simulink model "formation_planner_exp_cs"  (R2022b)
settings: Solver=ode5  StartTime=0.0  StopTime=80  FixedStep=1/1000  RelTol=1e-3
PreLoadFcn:
  | mbxruntime.callbacks.PreLoadFcn(bdroot);
PostLoadFcn:
  | mbxruntime.callbacks.PostLoadFcn(bdroot);
InitFcn:
  | mbxruntime.callbacks.InitFcn(bdroot);
StartFcn:
  | mbxruntime.callbacks.StartFcn(bdroot);
StopFcn:
  | mbxruntime.callbacks.StopFcn(bdroot);
model workspace (MAT data in the model file):
  mbox_table : object (value not decoded)
  model_closed = 0
  sim_status = 0
values from neighbouring files (symbols this model uses):
  c_factor = 43.75    [emplanner_init.m]
  car1_s = -10    [emplanner_init.m]
  car2_s = -20    [emplanner_init.m]
  cf = -175016    [emplanner_init.m]
  cr = -130634    [emplanner_init.m]
  KD_PID_distance = 0.0    (= 0)    [emplanner_init.m]
  KD_PID_speed = 0    [emplanner_init.m]
  KI_PID_distance = 0.0    (= 0)    [emplanner_init.m]
  KI_PID_speed = 0    [emplanner_init.m]
  KP_PID_distance = 0.5    [emplanner_init.m]
  KP_PID_speed = 1.8    [emplanner_init.m]
  la = 1.265    [emplanner_init.m]
  lb = 2.947-1.265    (= 1.682)    [emplanner_init.m]
  leader_global_kappa = global_kappa    [kappa.m]    (also in leader_global_path.mat = [0 0 0 0 0 0 0 0 0 0 0 0 ... (801 elements, 801x1)])
  leader_global_path_x = x_orgin.Data    [kappa.m]    (also in leader_global_path.mat = [2.22044604925e-16 0.999382255067 1.99750536558 2.9943522493)
  leader_global_path_y = y.Data    [kappa.m]    (also in leader_global_path.mat = [2 2 2 2 2 2 2 2 2 2 2 2 ... (801 elements, 801x1)])
  leader_global_yaw = yaw.Data    [kappa.m]    (also in leader_global_path.mat = [0 0 0 0 0 0 0 0 0 0 0 0 ... (801 elements, 801x1)])
  LQR_K1 = k(:,1)'    [emplanner_init.m]
  LQR_K2 = k(:,2)'    [emplanner_init.m]
  LQR_K3 = k(:,3)'    [emplanner_init.m]
  LQR_K4 = k(:,4)'    [emplanner_init.m]
  m = 2020    [emplanner_init.m]
  rack_displacement = [-39.14 , -37.2 , -35.29 , -33.43 , -31.6 , -29.81 , -28.06 , -26.34 , -24.66 ,      -23.01 , -21.38 , -19.79 , -18.23 , -16.69 , -15.18 , -13.7 , -12.23 , -10.8 , -9.38 , -7.98 ,     -6.61 , -5.25 , -3.91 , -2.59 , -1.29 , 0 , 1.27 , 2.54 , 3.78 , 5.02 , 6.24 , 7.46 , 8.66 ,      9.86 , 11.05 , 12.24 , 13.41 , 14.59 , 15.76 , 16.92 , 18.09 , 19.25 , 20.42 , 21.59 , 22.76 ,      23.93 , 25.11 , 26 ...(+26 chars)    [emplanner_init.m]
  right_wheel_ground = [-70 ,-67.2 , -64.4 , -61.6 , -58.8 , -56 , -53.2 , -50.4 , -47.6 , -44.8 , -42 ,      -39.2 , -36.4 , -33.6 , -30.8 , -28 , -25.2 , -22.4 , -19.6 , -16.8 , -14 , -11.2 , -8.4 , -5.6 ,      -2.8 , 0 , 2.8 , 5.6 , 8.4 , 11.2 , 14 , 16.8 , 19.6 , 22.4 , 25.2 , 28 , 30.8 , 33.6 , 36.4 ,      39.2 , 42 , 44.8 , 47.6 , 50.4 , 53.2 , 56 , 58.8 , 61.6 , 64.4 , 67.2 , 70 ]    [emplanner_init.m]
  vx_break_point = zeros(1,5000)    [emplanner_init.m]
undefined symbols (not defined in the file or in its folder): aubr, car1_global_kappa, car1_global_path_x, car1_global_path_y, car1_global_yaw, car2_global_kappa, car2_global_path_x, car2_global_path_y, car2_global_yaw, DiscIntNeverNeededParam, tablebr, vubr, warningInitialVelocity, x0
libraries: PreScanSimulinkLibrary x65, simulink x19, simulink_extras x14, Solver_SF x2
(part 15 of 31)

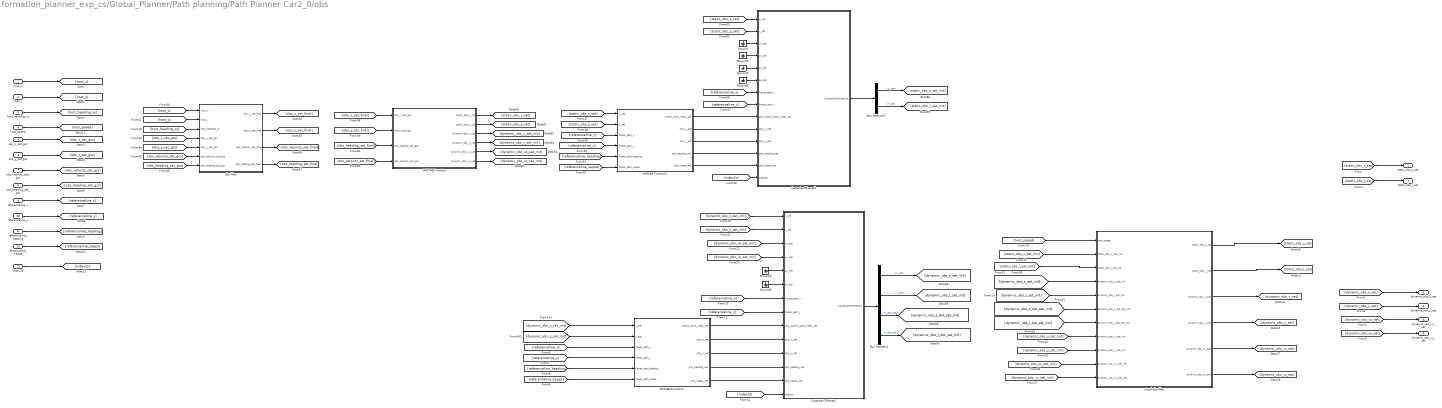
== system formation_planner_exp_cs/Global_Planner/Path planning/Path Planner Car2_0/obs ==
  host_x : Inport
  host_y : Inport  Port=2
  host_heading_xy : Inport  Port=3
  host_speed : Inport  Port=4
  obs_x_set_gcs : Inport  Port=5
  obs_y_set_gcs : Inport  Port=6
  obs_velocity_set_gcs : Inport  Port=7
  obs_heading_set_gcs : Inport  Port=8
  referenceline_x : Inport  Port=9
  referenceline_y : Inport  Port=10
  referenceline_heading : Inport  Port=11
  referenceline_kappa : Inport  Port=12
  index2s : Inport  Port=13
  Bus Selector1 : BusSelector  OutputSignals=s_set,l_set,s_dot_set,l_dot_set
  Bus Selector5 : BusSelector  OutputSignals=s_set,l_set
  Cartesian2Frenet1 : Subsystem
  Cartesian2Frenet2 : Subsystem
  Ground{,1..5} (6 alike) : Ground
  MATLAB Function : MATLAB Function  TreatAsAtomicUnit=on
  MATLAB Function1 : MATLAB Function  TreatAsAtomicUnit=on
  MATLAB Function2 : MATLAB Function  TreatAsAtomicUnit=on
  obs filter : MATLAB Function  TreatAsAtomicUnit=on
  visual obs filter : MATLAB Function  TreatAsAtomicUnit=on
  static_obs_s_set : Outport
  static_obs_l_set : Outport  Port=2
  dynamic_obs_x_set : Outport  Port=3
  dynamic_obs_y_set : Outport  Port=4
  dynamic_obs_vx_set : Outport  Port=5
  dynamic_obs_vy_set : Outport  Port=6
  wires:
  Ground3/1 -> Cartesian2Frenet1/6(ay_set)
  [obs_x_set_gcs] -> obs filter/4(obs_x_set_gcs)
  [index2s] -> Cartesian2Frenet1/14(index2s)
  [referenceline_y] -> Cartesian2Frenet1/8(frenet_path_y)
  MATLAB Function2/5(proj_kappa_set) -> Cartesian2Frenet1/13(proj_kappa_set)
  MATLAB Function2/4(proj_heading_set) -> Cartesian2Frenet1/12(proj_heading_set)
  [referenceline_x] -> MATLAB Function2/3(frenet_path_x)
  Ground2/1 -> Cartesian2Frenet1/5(ax_set)
  obs filter/1(obs_x_set_final) -> [obs_x_set_final]
  obs filter/4(obs_heading_set_final) -> [obs_heading_set_final]
  [host_heading_xy] -> obs filter/3(host_heading_xy)
  MATLAB Function/5(dynamic_obs_vx_set) -> [dynamic_obs_vx_set_init]
  [obs_y_set_final] -> MATLAB Function/2(obs_y_set_gcs)
  MATLAB Function/6(dynamic_obs_vy_set) -> [dynamic_obs_vy_set_init]
  [referenceline_y] -> MATLAB Function2/4(frenet_path_y)
  obs filter/3(obs_velocity_set_final) -> [obs_velocity_set_final]
  MATLAB Function/1(static_obs_x_set) -> [static_obs_x_set]
  [obs_heading_set_gcs] -> obs filter/7(obs_heading_set_gcs)
  [referenceline_kappa] -> MATLAB Function2/6(frenet_path_kappa)
  [static_obs_x_set] -> Cartesian2Frenet1/1(x_set)
  [static_obs_y_set] -> MATLAB Function2/2(y_set)
  [referenceline_x] -> Cartesian2Frenet1/7(frenet_path_x)
  Ground1/1 -> Cartesian2Frenet1/4(vy_set)
  [obs_x_set_final] -> MATLAB Function/1(obs_x_set_gcs)
  [obs_velocity_set_gcs] -> obs filter/6(obs_velocity_set_gcs)
  [host_y] -> obs filter/2(host_y)
  Bus Selector5/2 -> [static_obs_l_set_init]  "<l_set>"
  [referenceline_heading] -> MATLAB Function2/5(frenet_path_heading)
  obs filter/2(obs_y_set_final) -> [obs_y_set_final]
  Bus Selector5/1 -> [static_obs_s_set_init]  "<s_set>"
  MATLAB Function/3(dynamic_obs_x_set) -> [dynamic_obs_x_set_init]
  MATLAB Function2/2(proj_x_set) -> Cartesian2Frenet1/10(proj_x_set)
  Ground/1 -> Cartesian2Frenet1/3(vx_set)
  MATLAB Function2/3(proj_y_set) -> Cartesian2Frenet1/11(proj_y_set)
  MATLAB Function/4(dynamic_obs_y_set) -> [dynamic_obs_y_set_init]
  MATLAB Function2/1(match_point_index_set) -> Cartesian2Frenet1/9(proj_match_point_index_set)
  [host_x] -> obs filter/1(host_x)
  [obs_y_set_gcs] -> obs filter/5(obs_y_set_gcs)
  Cartesian2Frenet1/1(Cartesian2FrenetOut) -> Bus Selector5/1
  [static_obs_x_set] -> MATLAB Function2/1(x_set)
  MATLAB Function/2(static_obs_y_set) -> [static_obs_y_set]
  [static_obs_y_set] -> Cartesian2Frenet1/2(y_set)
  host_x/1 -> [host_x]
  host_y/1 -> [host_y]
  host_heading_xy/1 -> [host_heading_xy]
  obs_x_set_gcs/1 -> [obs_x_set_gcs]
  obs_y_set_gcs/1 -> [obs_y_set_gcs]
  obs_velocity_set_gcs/1 -> [obs_velocity_set_gcs]
  obs_heading_set_gcs/1 -> [obs_heading_set_gcs]
  referenceline_x/1 -> [referenceline_x]
  referenceline_y/1 -> [referenceline_y]
  referenceline_heading/1 -> [referenceline_heading]
  referenceline_kappa/1 -> [referenceline_kappa]
  index2s/1 -> [index2s]
  [static_obs_s_set] -> static_obs_s_set/1
  [static_obs_l_set] -> static_obs_l_set/1
  [dynamic_obs_vy_set] -> dynamic_obs_vy_set/1
  [dynamic_obs_vx_set] -> dynamic_obs_vx_set/1
  [dynamic_obs_y_set] -> dynamic_obs_y_set/1
  [dynamic_obs_x_set] -> dynamic_obs_x_set/1
  [obs_velocity_set_final] -> MATLAB Function/4(obs_velocity_set_gcs)
  [obs_heading_set_final] -> MATLAB Function/3(obs_heading_set_gcs)
  [referenceline_x] -> Cartesian2Frenet2/7(frenet_path_x)
  Bus Selector1/1 -> [dynamic_obs_s_set_init]  "<s_set>"
  Ground4/1 -> Cartesian2Frenet2/5(ax_set)
  MATLAB Function1/2(proj_x_set) -> Cartesian2Frenet2/10(proj_x_set)
  Bus Selector1/2 -> [dynamic_obs_l_set_init]  "<l_set>"
  [dynamic_obs_vx_set_init] -> Cartesian2Frenet2/3(vx_set)
  [dynamic_obs_y_set_init] -> MATLAB Function1/2(y_set)
  Bus Selector1/4 -> [dynamic_obs_l_dot_set_init]  "<l_dot_set>"
  [referenceline_kappa] -> MATLAB Function1/6(frenet_path_kappa)
  Cartesian2Frenet2/1(Cartesian2FrenetOut) -> Bus Selector1/1
  MATLAB Function1/3(proj_y_set) -> Cartesian2Frenet2/11(proj_y_set)
  [index2s] -> Cartesian2Frenet2/14(index2s)
  MATLAB Function1/1(match_point_index_set) -> Cartesian2Frenet2/9(proj_match_point_index_set)
  [referenceline_heading] -> MATLAB Function1/5(frenet_path_heading)
  [dynamic_obs_y_set_init] -> Cartesian2Frenet2/2(y_set)
  [dynamic_obs_vy_set_init] -> Cartesian2Frenet2/4(vy_set)
  [referenceline_y] -> Cartesian2Frenet2/8(frenet_path_y)
  [referenceline_y] -> MATLAB Function1/4(frenet_path_y)
  [dynamic_obs_x_set_init] -> MATLAB Function1/1(x_set)
  Bus Selector1/3 -> [dynamic_obs_s_dot_set_init]  "<s_dot_set>"
  MATLAB Function1/4(proj_heading_set) -> Cartesian2Frenet2/12(proj_heading_set)
  Ground5/1 -> Cartesian2Frenet2/6(ay_set)
  [dynamic_obs_x_set_init] -> Cartesian2Frenet2/1(x_set)
  MATLAB Function1/5(proj_kappa_set) -> Cartesian2Frenet2/13(proj_kappa_set)
  [referenceline_x] -> MATLAB Function1/3(frenet_path_x)
  [dynamic_obs_s_dot_set_init] -> visual obs filter/6(dynamic_obs_s_dot_set_init)
  [dynamic_obs_l_dot_set_init] -> visual obs filter/7(dynamic_obs_l_dot_set_init)
  [dynamic_obs_s_set_init] -> visual obs filter/4(dynamic_obs_s_set_init)
  [dynamic_obs_l_set_init] -> visual obs filter/5(dynamic_obs_l_set_init)
  [static_obs_s_set_init] -> visual obs filter/2(static_obs_s_set_init)
  [static_obs_l_set_init] -> visual obs filter/3(static_obs_l_set_init)
  host_speed/1 -> [host_speed]
  [host_speed] -> visual obs filter/1(host_speed)
  visual obs filter/6(dynamic_obs_vy_set) -> [dynamic_obs_vy_set]
  visual obs filter/5(dynamic_obs_vx_set) -> [dynamic_obs_vx_set]
  visual obs filter/4(dynamic_obs_y_set) -> [dynamic_obs_y_set]
  visual obs filter/1(static_obs_s_set) -> [static_obs_s_set]
  visual obs filter/2(static_obs_l_set) -> [static_obs_l_set]
  visual obs filter/3(dynamic_obs_x_set) -> [dynamic_obs_x_set]
  [dynamic_obs_x_set_init] -> visual obs filter/8(dynamic_obs_x_set_init)
  [dynamic_obs_y_set_init] -> visual obs filter/9(dynamic_obs_y_set_init)
  [dynamic_obs_vx_set_init] -> visual obs filter/10(dynamic_obs_vx_set_init)
  [dynamic_obs_vy_set_init] -> visual obs filter/11(dynamic_obs_vy_set_init)

== system formation_planner_exp_cs/Global_Planner/Path planning/Path Planner Car2_0/path decision task ==
  static_obs_s_set : Inport
  static_obs_l_set : Inport  Port=2
  plan_start_s : Inport  Port=3
  plan_start_l : Inport  Port=4
  plan_start_dl : Inport  Port=5
  plan_start_ddl : Inport  Port=6
  dp_cost_collision : Inport  Port=7
  dp_cost_dl : Inport  Port=8
  dp_cost_ddl : Inport  Port=9
  dp_cost_dddl : Inport  Port=10
  dp_cost_ref : Inport  Port=11
  dp_row : Inport  Port=12
  dp_col : Inport  Port=13
  dp_sample_s : Inport  Port=14
  dp_sample_l : Inport  Port=15
  increase DP path nodes : MATLAB Function  TreatAsAtomicUnit=on
  path decision with dynamic planning(dp) : MATLAB Function  TreatAsAtomicUnit=on
  dp_path_s_final : Outport
  dp_path_l_final : Outport  Port=2
  dp_path_dl_final : Outport  Port=3
  dp_path_ddl_final : Outport  Port=4
  wires:
  [plan_start_s] -> path decision with dynamic planning(dp)/3(plan_start_s)
  path decision with dynamic planning(dp)/1(dp_path_s) -> [dp_path_s_init]
  increase DP path nodes/2(dp_path_l_final) -> [dp_path_l_final]
  [static_obs_l_set] -> path decision with dynamic planning(dp)/2(obs_l_set)
  [plan_start_ddl] -> path decision with dynamic planning(dp)/6(plan_start_dll)
  [plan_start_l] -> path decision with dynamic planning(dp)/4(plan_start_l)
  [static_obs_s_set] -> path decision with dynamic planning(dp)/1(obs_s_set)
  [plan_start_dl] -> increase DP path nodes/5(plan_start_dl)
  increase DP path nodes/4(dp_path_ddl_final) -> [dp_path_ddl_final]
  increase DP path nodes/1(dp_path_s_final) -> [dp_path_s_final]
  increase DP path nodes/3(dp_path_dl_final) -> [dp_path_dl_final]
  path decision with dynamic planning(dp)/2(dp_path_l) -> [dp_path_l_init]
  [plan_start_l] -> increase DP path nodes/4(plan_start_l)
  [plan_start_ddl] -> increase DP path nodes/6(plan_start_ddl)
  [plan_start_dl] -> path decision with dynamic planning(dp)/5(plan_start_dl)
  [plan_start_s] -> increase DP path nodes/3(plan_start_s)
  [dp_path_l_init] -> increase DP path nodes/2(dp_path_l_init)
  [dp_path_s_init] -> increase DP path nodes/1(dp_path_s_init)
  static_obs_s_set/1 -> [static_obs_s_set]
  static_obs_l_set/1 -> [static_obs_l_set]
  plan_start_s/1 -> [plan_start_s]
  plan_start_l/1 -> [plan_start_l]
  plan_start_dl/1 -> [plan_start_dl]
  plan_start_ddl/1 -> [plan_start_ddl]
  [dp_path_s_final] -> dp_path_s_final/1
  [dp_path_l_final] -> dp_path_l_final/1
  [dp_path_dl_final] -> dp_path_dl_final/1
  [dp_path_ddl_final] -> dp_path_ddl_final/1
  [dp_cost_collision] -> path decision with dynamic planning(dp)/7(w_cost_collision)
  [dp_cost_dl] -> path decision with dynamic planning(dp)/8(w_cost_smooth_dl)
  [dp_cost_ddl] -> path decision with dynamic planning(dp)/9(w_cost_smooth_ddl)
  [dp_cost_dddl] -> path decision with dynamic planning(dp)/10(w_cost_smooth_dddl)
  [dp_cost_ref] -> path decision with dynamic planning(dp)/11(w_cost_ref)
  [dp_row] -> path decision with dynamic planning(dp)/12(row)
  [dp_col] -> path decision with dynamic planning(dp)/13(col)
  [dp_sample_s] -> path decision with dynamic planning(dp)/14(sample_s)
  [dp_sample_l] -> path decision with dynamic planning(dp)/15(sample_l)
  dp_cost_dl/1 -> [dp_cost_dl]
  dp_cost_ddl/1 -> [dp_cost_ddl]
  dp_cost_dddl/1 -> [dp_cost_dddl]
  dp_cost_ref/1 -> [dp_cost_ref]
  dp_row/1 -> [dp_row]
  dp_col/1 -> [dp_col]
  dp_sample_l/1 -> [dp_sample_l]
  dp_sample_s/1 -> [dp_sample_s]
  dp_cost_collision/1 -> [dp_cost_collision]

== system formation_planner_exp_cs/Global_Planner/Path planning/Path Planner Car2_0/path planning task ==
  dp_path_s_final : Inport
  dp_path_l_final : Inport  Port=2
  static_obs_s_set : Inport  Port=3
  static_obs_l_set : Inport  Port=4
  plan_start_s : Inport  Port=5
  plan_start_l : Inport  Port=6
  plan_start_dl : Inport  Port=7
  plan_start_ddl : Inport  Port=8
  qp_cost_l : Inport  Port=9
  qp_cost_dl : Inport  Port=10
  qp_cost_ddl : Inport  Port=11
  qp_cost_dddl : Inport  Port=12
  qp_cost_centre : Inport  Port=13
  qp_cost_endl : Inport  Port=14
  qp_cost_end_dl : Inport  Port=15
  qp_cost_end_ddl : Inport  Port=16
  host_d1 : Inport  Port=17
  host_d2 : Inport  Port=18
  host_w : Inport  Port=19
  delta_dl_max : Inport  Port=20
  delta_ddl_max : Inport  Port=21
  Constant10 : Constant  Value=5
  Constant11 : Constant  Value=3
  MATLAB Function : MATLAB Function  TreatAsAtomicUnit=on
  generate convex space : MATLAB Function  TreatAsAtomicUnit=on
  path planning with quadratic programming (qp) : MATLAB Function  TreatAsAtomicUnit=on
  qp_path_s_final : Outport
  qp_path_l_final : Outport  Port=2
  qp_path_dl_final : Outport  Port=3
  qp_path_ddl_final : Outport  Port=4
  wires:
  generate convex space/2(l_max) -> [l_max]
  Constant11/1 -> generate convex space/6(static_obs_width)
  Constant10/1 -> generate convex space/5(static_obs_length)
  [static_obs_l_set] -> generate convex space/4(static_obs_l_set)
  [dp_path_s_final] -> generate convex space/1(dp_path_s)
  [plan_start_l] -> path planning with quadratic programming (qp)/15(plan_start_l)
  generate convex space/1(l_min) -> [l_min]
  [static_obs_s_set] -> generate convex space/3(static_obs_s_set)
  [dp_path_l_final] -> generate convex space/2(dp_path_l)
  [plan_start_dl] -> path planning with quadratic programming (qp)/16(plan_start_dl)
  [l_max] -> path planning with quadratic programming (qp)/2(l_max)
  [l_min] -> path planning with quadratic programming (qp)/1(l_min)
  [plan_start_ddl] -> path planning with quadratic programming (qp)/17(plan_start_ddl)
  dp_path_s_final/1 -> [dp_path_s_final]
  dp_path_l_final/1 -> [dp_path_l_final]
  static_obs_s_set/1 -> [static_obs_s_set]
  static_obs_l_set/1 -> [static_obs_l_set]
  plan_start_l/1 -> [plan_start_l]
  plan_start_dl/1 -> [plan_start_dl]
  plan_start_ddl/1 -> [plan_start_ddl]
  [qp_cost_l] -> path planning with quadratic programming (qp)/3(w_cost_l)
  [qp_cost_dl] -> path planning with quadratic programming (qp)/4(w_cost_dl)
  [qp_cost_ddl] -> path planning with quadratic programming (qp)/5(w_cost_ddl)
  [qp_cost_dddl] -> path planning with quadratic programming (qp)/6(w_cost_dddl)
  [qp_cost_centre] -> path planning with quadratic programming (qp)/7(w_cost_centre)
  [qp_cost_endl] -> path planning with quadratic programming (qp)/8(w_cost_end_l)
  [qp_cost_end_dl] -> path planning with quadratic programming (qp)/9(w_cost_end_dl)
  [qp_cost_end_ddl] -> path planning with quadratic programming (qp)/10(w_cost_end_ddl)
  [host_d1] -> path planning with quadratic programming (qp)/11(host_d1)
  [host_d2] -> path planning with quadratic programming (qp)/12(host_d2)
  [host_w] -> path planning with quadratic programming (qp)/13(host_w)
  qp_cost_l/1 -> [qp_cost_l]
  qp_cost_dl/1 -> [qp_cost_dl]
  qp_cost_ddl/1 -> [qp_cost_ddl]
  qp_cost_dddl/1 -> [qp_cost_dddl]
  qp_cost_centre/1 -> [qp_cost_centre]
  qp_cost_endl/1 -> [qp_cost_endl]
  qp_cost_end_dl/1 -> [qp_cost_end_dl]
  qp_cost_end_ddl/1 -> [qp_cost_end_ddl]
  host_d1/1 -> [host_d1]
  host_d2/1 -> [host_d2]
  host_w/1 -> [host_w]
  [delta_dl_max] -> path planning with quadratic programming (qp)/18(delta_dl_max)
  [delta_ddl_max] -> path planning with quadratic programming (qp)/19(delta_ddl_max)
  delta_dl_max/1 -> [delta_dl_max]
  delta_ddl_max/1 -> [delta_ddl_max]
  plan_start_s/1 -> [plan_start_s]
  [plan_start_s] -> path planning with quadratic programming (qp)/14(plan_start_s)
  MATLAB Function/1(qp_path_s_final) -> [qp_path_s_final]
  MATLAB Function/3(qp_path_dl_final) -> [qp_path_dl_final]
  [qp_path_s] -> MATLAB Function/1(qp_path_s)
  [qp_path_ddl] -> MATLAB Function/4(qp_path_ddl)
  MATLAB Function/2(qp_path_l_final) -> [qp_path_l_final]
  [qp_path_dl] -> MATLAB Function/3(qp_path_dl)
  MATLAB Function/4(qp_path_ddl_final) -> [qp_path_ddl_final]
  [qp_path_l] -> MATLAB Function/2(qp_path_l)
  [qp_path_s_final] -> qp_path_s_final/1
  [qp_path_l_final] -> qp_path_l_final/1
  [qp_path_dl_final] -> qp_path_dl_final/1
  [qp_path_ddl_final] -> qp_path_ddl_final/1
  path planning with quadratic programming (qp)/1(qp_path_s) -> [qp_path_s]
  path planning with quadratic programming (qp)/2(qp_path_l) -> [qp_path_l]
  path planning with quadratic programming (qp)/3(qp_path_dl) -> [qp_path_dl]
  path planning with quadratic programming (qp)/4(qp_path_ddl) -> [qp_path_ddl]

== system formation_planner_exp_cs/Global_Planner/Path planning/Planner Car1/Cartesian2Frenet ==
  x_set : Inport
  y_set : Inport  Port=2
  vx_set : Inport  Port=3
  vy_set : Inport  Port=4
  ax_set : Inport  Port=5
  ay_set : Inport  Port=6
  frenet_path_x : Inport  Port=7
  frenet_path_y : Inport  Port=8
  proj_match_point_index_set : Inport  Port=9
  proj_x_set : Inport  Port=10
  proj_y_set : Inport  Port=11
  proj_heading_set : Inport  Port=12
  proj_kappa_set : Inport  Port=13
  index2s : Inport  Port=14
  Bus Creator : BusCreator  Inputs=8
  MATLAB Function : MATLAB Function  TreatAsAtomicUnit=on
  MATLAB Function1 : MATLAB Function  TreatAsAtomicUnit=on
  MATLAB Function2 : MATLAB Function  TreatAsAtomicUnit=on
  Cartesian2FrenetOut : Outport
  wires:
  Bus Creator/1 -> Cartesian2FrenetOut/1
  [ddl_set] -> Bus Creator/8  "ddl_set"
  [l_dot2_set] -> Bus Creator/7  "l_dot2_set"
  [s_dot2_set] -> Bus Creator/6  "s_dot2_set"
  [dl_set] -> Bus Creator/5  "dl_set"
  [l_dot_set] -> Bus Creator/4  "l_dot_set"
  [s_dot_set] -> Bus Creator/3  "s_dot_set"
  [l_set] -> Bus Creator/2  "l_set"
  [s_set] -> Bus Creator/1  "s_set"
  MATLAB Function2/3(ddl_set) -> [ddl_set]
  MATLAB Function2/2(l_dot2_set) -> [l_dot2_set]
  MATLAB Function2/1(s_dot2_set) -> [s_dot2_set]
  [dl_set] -> MATLAB Function2/7(dl_set)
  [s_dot_set] -> MATLAB Function2/6(s_dot_set)
  MATLAB Function1/3(dl_set) -> [dl_set]
  MATLAB Function1/2(l_dot_set) -> [l_dot_set]
  MATLAB Function1/1(s_dot_set) -> [s_dot_set]
  [l_set] -> MATLAB Function2/5(l_set)
  [proj_kappa_set] -> MATLAB Function2/4(proj_kappa_set)
  [proj_heading_set] -> MATLAB Function2/3(proj_heading_set)
  [ay_set] -> MATLAB Function2/2(ay_set)
  [ax_set] -> MATLAB Function2/1(ax_set)
  [proj_kappa_set] -> MATLAB Function1/5(proj_kappa_set)
  [proj_heading_set] -> MATLAB Function1/4(proj_heading_set)
  [vy_set] -> MATLAB Function1/3(vy_set)
  [vx_set] -> MATLAB Function1/2(vx_set)
  [l_set] -> MATLAB Function1/1(l_set)
  MATLAB Function/2(l_set) -> [l_set]
  MATLAB Function/1(s_set) -> [s_set]
  [index2s] -> MATLAB Function/9(index2s)
  [proj_heading_set] -> MATLAB Function/7(proj_heading_set)
  [proj_y_set] -> MATLAB Function/6(proj_y_set)
  [proj_match_point_index_set] -> MATLAB Function/8(proj_match_point_index_set)
  [proj_x_set] -> MATLAB Function/5(proj_x_set)
  [frenet_path_y] -> MATLAB Function/4(frenet_path_y)
  [frenet_path_x] -> MATLAB Function/3(frenet_path_x)
  [y_set] -> MATLAB Function/2(y_set)
  [x_set] -> MATLAB Function/1(x_set)
  index2s/1 -> [index2s]
  proj_kappa_set/1 -> [proj_kappa_set]
  proj_heading_set/1 -> [proj_heading_set]
  proj_y_set/1 -> [proj_y_set]
  proj_x_set/1 -> [proj_x_set]
  proj_match_point_index_set/1 -> [proj_match_point_index_set]
  frenet_path_y/1 -> [frenet_path_y]
  frenet_path_x/1 -> [frenet_path_x]
  ay_set/1 -> [ay_set]
  ax_set/1 -> [ax_set]
  vy_set/1 -> [vy_set]
  vx_set/1 -> [vx_set]
  y_set/1 -> [y_set]
  x_set/1 -> [x_set]

== system formation_planner_exp_cs/Global_Planner/Path planning/Planner Car1/Cartesian2Frenet1 ==
  x_set : Inport
  y_set : Inport  Port=2
  vx_set : Inport  Port=3
  vy_set : Inport  Port=4
  ax_set : Inport  Port=5
  ay_set : Inport  Port=6
  frenet_path_x : Inport  Port=7
  frenet_path_y : Inport  Port=8
  proj_match_point_index_set : Inport  Port=9
  proj_x_set : Inport  Port=10
  proj_y_set : Inport  Port=11
  proj_heading_set : Inport  Port=12
  proj_kappa_set : Inport  Port=13
  index2s : Inport  Port=14
  Bus Creator : BusCreator  Inputs=8
  From14 : From  Commented=on  GotoTag=ax_set
  From15 : From  Commented=on  GotoTag=ay_set
  From16 : From  Commented=on  GotoTag=proj_heading_set
  From17 : From  Commented=on  GotoTag=proj_kappa_set
  From18 : From  Commented=on  GotoTag=l_set
  From19 : From  Commented=on  GotoTag=s_dot_set
  From20 : From  Commented=on  GotoTag=dl_set
  Goto19 : Goto  Commented=on  GotoTag=s_dot2_set
  Goto20 : Goto  Commented=on  GotoTag=l_dot2_set
  Goto21 : Goto  Commented=on  GotoTag=ddl_set
  MATLAB Function : MATLAB Function  TreatAsAtomicUnit=on
  MATLAB Function1 : MATLAB Function  TreatAsAtomicUnit=on
  MATLAB Function2 : MATLAB Function  Commented=on  TreatAsAtomicUnit=on
  Cartesian2FrenetOut : Outport
  wires:
  x_set/1 -> [x_set]
  y_set/1 -> [y_set]
  vx_set/1 -> [vx_set]
  vy_set/1 -> [vy_set]
  ax_set/1 -> [ax_set]
  ay_set/1 -> [ay_set]
  frenet_path_x/1 -> [frenet_path_x]
  frenet_path_y/1 -> [frenet_path_y]
  proj_match_point_index_set/1 -> [proj_match_point_index_set]
  proj_x_set/1 -> [proj_x_set]
  proj_y_set/1 -> [proj_y_set]
  proj_heading_set/1 -> [proj_heading_set]
  proj_kappa_set/1 -> [proj_kappa_set]
  index2s/1 -> [index2s]
  [x_set] -> MATLAB Function/1(x_set)
  [y_set] -> MATLAB Function/2(y_set)
  [frenet_path_x] -> MATLAB Function/3(frenet_path_x)
  [frenet_path_y] -> MATLAB Function/4(frenet_path_y)
  [proj_x_set] -> MATLAB Function/5(proj_x_set)
  [proj_match_point_index_set] -> MATLAB Function/8(proj_match_point_index_set)
  [proj_y_set] -> MATLAB Function/6(proj_y_set)
  [proj_heading_set] -> MATLAB Function/7(proj_heading_set)
  [index2s] -> MATLAB Function/9(index2s)
  MATLAB Function/1(s_set) -> [s_set]
  MATLAB Function/2(l_set) -> [l_set]
  [l_set] -> MATLAB Function1/1(l_set)
  [vx_set] -> MATLAB Function1/2(vx_set)
  [vy_set] -> MATLAB Function1/3(vy_set)
  [proj_heading_set] -> MATLAB Function1/4(proj_heading_set)
  [proj_kappa_set] -> MATLAB Function1/5(proj_kappa_set)
  From14/1 -> MATLAB Function2/1(ax_set)
  From15/1 -> MATLAB Function2/2(ay_set)
  From16/1 -> MATLAB Function2/3(proj_heading_set)
  From17/1 -> MATLAB Function2/4(proj_kappa_set)
  From18/1 -> MATLAB Function2/5(l_set)
  MATLAB Function1/1(s_dot_set) -> [s_dot_set]
  MATLAB Function1/2(l_dot_set) -> [l_dot_set]
  MATLAB Function1/3(dl_set) -> [dl_set]
  From19/1 -> MATLAB Function2/6(s_dot_set)
  From20/1 -> MATLAB Function2/7(dl_set)
  MATLAB Function2/1(s_dot2_set) -> Goto19/1
  MATLAB Function2/2(l_dot2_set) -> Goto20/1
  MATLAB Function2/3(ddl_set) -> Goto21/1
  [s_set] -> Bus Creator/1  "s_set"
  [l_set] -> Bus Creator/2  "l_set"
  [s_dot_set] -> Bus Creator/3  "s_dot_set"
  [l_dot_set] -> Bus Creator/4  "l_dot_set"
  [dl_set] -> Bus Creator/5  "dl_set"
  [s_dot2_set] -> Bus Creator/6  "s_dot2_set"
  [l_dot2_set] -> Bus Creator/7  "l_dot2_set"
  [ddl_set] -> Bus Creator/8  "ddl_set"
  Bus Creator/1 -> Cartesian2FrenetOut/1

== system formation_planner_exp_cs/Global_Planner/Path planning/Planner Car1/Cartesian2Frenet2 ==
  x_set : Inport
  y_set : Inport  Port=2
  vx_set : Inport  Port=3
  vy_set : Inport  Port=4
  ax_set : Inport  Port=5
  ay_set : Inport  Port=6
  frenet_path_x : Inport  Port=7
  frenet_path_y : Inport  Port=8
  proj_match_point_index_set : Inport  Port=9
  proj_x_set : Inport  Port=10
  proj_y_set : Inport  Port=11
  proj_heading_set : Inport  Port=12
  proj_kappa_set : Inport  Port=13
  index2s : Inport  Port=14
  Bus Creator : BusCreator  Inputs=8
  From10 : From  Commented=on  GotoTag=vx_set
  From11 : From  Commented=on  GotoTag=vy_set
  From12 : From  Commented=on  GotoTag=proj_heading_set
  From13 : From  Commented=on  GotoTag=proj_kappa_set
  From14 : From  Commented=on  GotoTag=ax_set
  From15 : From  Commented=on  GotoTag=ay_set
  From16 : From  Commented=on  GotoTag=proj_heading_set
  From17 : From  Commented=on  GotoTag=proj_kappa_set
  From18 : From  Commented=on  GotoTag=l_set
  From19 : From  Commented=on  GotoTag=s_dot_set
  From20 : From  Commented=on  GotoTag=dl_set
  From7 : From  Commented=on  GotoTag=l_set
  MATLAB Function : MATLAB Function  TreatAsAtomicUnit=on
  MATLAB Function1 : MATLAB Function  Commented=on  TreatAsAtomicUnit=on
  MATLAB Function2 : MATLAB Function  Commented=on  TreatAsAtomicUnit=on
  Selector1 : Selector  InputPortWidth=128  IndexOptions=Index vector (dialog)  Indices=1  OutputSizes=1
  Selector5 : Selector  InputPortWidth=128  IndexOptions=Index vector (dialog)  Indices=1  OutputSizes=1
  Cartesian2FrenetOut : Outport
  wires:
  Selector1/1 -> Bus Creator/2  "l_set"
  [l_set] -> Selector1/1  "l_set"
  Selector5/1 -> Bus Creator/1  "s_set"
  [s_set] -> Selector5/1  "s_set"
  x_set/1 -> [x_set]
  y_set/1 -> [y_set]
  vx_set/1 -> [vx_set]
  vy_set/1 -> [vy_set]
  ax_set/1 -> [ax_set]
  ay_set/1 -> [ay_set]
  frenet_path_x/1 -> [frenet_path_x]
  frenet_path_y/1 -> [frenet_path_y]
  proj_match_point_index_set/1 -> [proj_match_point_index_set]
  proj_x_set/1 -> [proj_x_set]
  proj_y_set/1 -> [proj_y_set]
  proj_heading_set/1 -> [proj_heading_set]
  proj_kappa_set/1 -> [proj_kappa_set]
  index2s/1 -> [index2s]
  [x_set] -> MATLAB Function/1(x_set)
  [y_set] -> MATLAB Function/2(y_set)
  [frenet_path_x] -> MATLAB Function/3(frenet_path_x)
  [frenet_path_y] -> MATLAB Function/4(frenet_path_y)
  [proj_x_set] -> MATLAB Function/5(proj_x_set)
  [proj_match_point_index_set] -> MATLAB Function/8(proj_match_point_index_set)
  [proj_y_set] -> MATLAB Function/6(proj_y_set)
  [proj_heading_set] -> MATLAB Function/7(proj_heading_set)
  [index2s] -> MATLAB Function/9(index2s)
  MATLAB Function/1(s_set) -> [s_set]
  MATLAB Function/2(l_set) -> [l_set]
  From7/1 -> MATLAB Function1/1(l_set)
  From10/1 -> MATLAB Function1/2(vx_set)
  From11/1 -> MATLAB Function1/3(vy_set)
  From12/1 -> MATLAB Function1/4(proj_heading_set)
  From13/1 -> MATLAB Function1/5(proj_kappa_set)
  From14/1 -> MATLAB Function2/1(ax_set)
  From15/1 -> MATLAB Function2/2(ay_set)
  From16/1 -> MATLAB Function2/3(proj_heading_set)
  From17/1 -> MATLAB Function2/4(proj_kappa_set)
  From18/1 -> MATLAB Function2/5(l_set)
  MATLAB Function1/1(s_dot_set) -> [s_dot_set]
  MATLAB Function1/2(l_dot_set) -> [l_dot_set]
  MATLAB Function1/3(dl_set) -> [dl_set]
  From19/1 -> MATLAB Function2/6(s_dot_set)
  From20/1 -> MATLAB Function2/7(dl_set)
  MATLAB Function2/1(s_dot2_set) -> [s_dot2_set]
  MATLAB Function2/2(l_dot2_set) -> [l_dot2_set]
  MATLAB Function2/3(ddl_set) -> [ddl_set]
  [s_dot_set] -> Bus Creator/3  "s_dot_set"
  [l_dot_set] -> Bus Creator/4  "l_dot_set"
  [dl_set] -> Bus Creator/5  "dl_set"
  [s_dot2_set] -> Bus Creator/6  "s_dot2_set"
  [l_dot2_set] -> Bus Creator/7  "l_dot2_set"
  [ddl_set] -> Bus Creator/8  "ddl_set"
  Bus Creator/1 -> Cartesian2FrenetOut/1

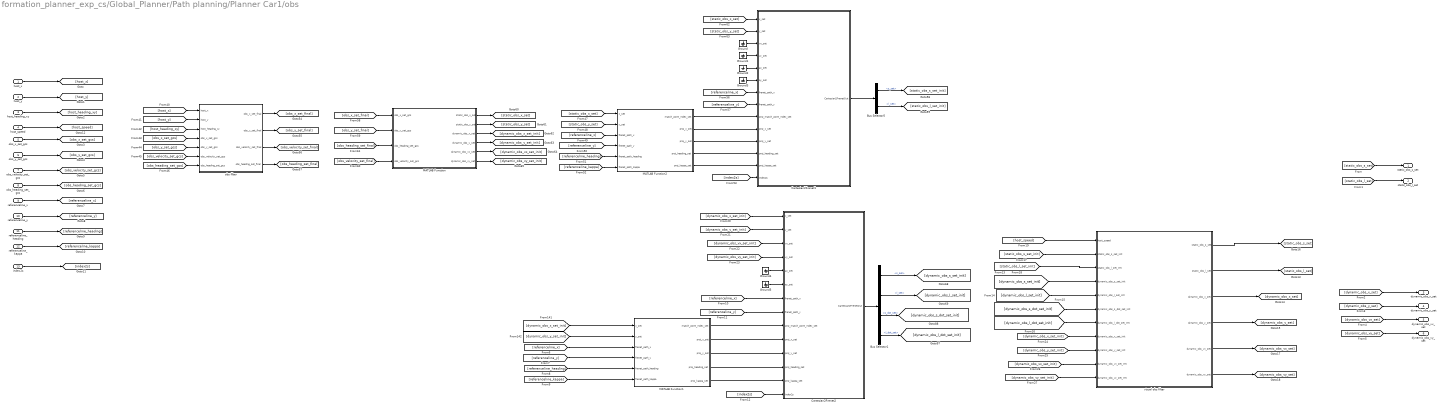
== system formation_planner_exp_cs/Global_Planner/Path planning/Planner Car1/obs ==
  host_x : Inport
  host_y : Inport  Port=2
  host_heading_xy : Inport  Port=3
  host_speed : Inport  Port=4
  obs_x_set_gcs : Inport  Port=5
  obs_y_set_gcs : Inport  Port=6
  obs_velocity_set_gcs : Inport  Port=7
  obs_heading_set_gcs : Inport  Port=8
  referenceline_x : Inport  Port=9
  referenceline_y : Inport  Port=10
  referenceline_heading : Inport  Port=11
  referenceline_kappa : Inport  Port=12
  index2s : Inport  Port=13
  Bus Selector1 : BusSelector  OutputSignals=s_set,l_set,s_dot_set,l_dot_set
  Bus Selector5 : BusSelector  OutputSignals=s_set,l_set
  Cartesian2Frenet1 : Subsystem
  Cartesian2Frenet2 : Subsystem
  Ground{,1..5} (6 alike) : Ground
  MATLAB Function : MATLAB Function  TreatAsAtomicUnit=on
  MATLAB Function1 : MATLAB Function  TreatAsAtomicUnit=on
  MATLAB Function2 : MATLAB Function  TreatAsAtomicUnit=on
  obs filter : MATLAB Function  TreatAsAtomicUnit=on
  visual obs filter : MATLAB Function  TreatAsAtomicUnit=on
  static_obs_s_set : Outport
  static_obs_l_set : Outport  Port=2
  dynamic_obs_x_set : Outport  Port=3
  dynamic_obs_y_set : Outport  Port=4
  dynamic_obs_vx_set : Outport  Port=5
  dynamic_obs_vy_set : Outport  Port=6
  wires:
  [dynamic_obs_vy_set_init] -> visual obs filter/11(dynamic_obs_vy_set_init)
  [dynamic_obs_vx_set_init] -> visual obs filter/10(dynamic_obs_vx_set_init)
  [dynamic_obs_y_set_init] -> visual obs filter/9(dynamic_obs_y_set_init)
  [dynamic_obs_x_set_init] -> visual obs filter/8(dynamic_obs_x_set_init)
  visual obs filter/3(dynamic_obs_x_set) -> [dynamic_obs_x_set]
  visual obs filter/2(static_obs_l_set) -> [static_obs_l_set]
  visual obs filter/1(static_obs_s_set) -> [static_obs_s_set]
  visual obs filter/4(dynamic_obs_y_set) -> [dynamic_obs_y_set]
  visual obs filter/5(dynamic_obs_vx_set) -> [dynamic_obs_vx_set]
  visual obs filter/6(dynamic_obs_vy_set) -> [dynamic_obs_vy_set]
  [host_speed] -> visual obs filter/1(host_speed)
  host_speed/1 -> [host_speed]
  [static_obs_l_set_init] -> visual obs filter/3(static_obs_l_set_init)
  [static_obs_s_set_init] -> visual obs filter/2(static_obs_s_set_init)
  [dynamic_obs_l_set_init] -> visual obs filter/5(dynamic_obs_l_set_init)
  [dynamic_obs_s_set_init] -> visual obs filter/4(dynamic_obs_s_set_init)
  [dynamic_obs_l_dot_set_init] -> visual obs filter/7(dynamic_obs_l_dot_set_init)
  [dynamic_obs_s_dot_set_init] -> visual obs filter/6(dynamic_obs_s_dot_set_init)
  [referenceline_x] -> MATLAB Function1/3(frenet_path_x)
  MATLAB Function1/5(proj_kappa_set) -> Cartesian2Frenet2/13(proj_kappa_set)
  [dynamic_obs_x_set_init] -> Cartesian2Frenet2/1(x_set)
  Ground5/1 -> Cartesian2Frenet2/6(ay_set)
  MATLAB Function1/4(proj_heading_set) -> Cartesian2Frenet2/12(proj_heading_set)
  Bus Selector1/3 -> [dynamic_obs_s_dot_set_init]  "<s_dot_set>"
  [dynamic_obs_x_set_init] -> MATLAB Function1/1(x_set)
  [referenceline_y] -> MATLAB Function1/4(frenet_path_y)
  [referenceline_y] -> Cartesian2Frenet2/8(frenet_path_y)
  [dynamic_obs_vy_set_init] -> Cartesian2Frenet2/4(vy_set)
  [dynamic_obs_y_set_init] -> Cartesian2Frenet2/2(y_set)
  [referenceline_heading] -> MATLAB Function1/5(frenet_path_heading)
  MATLAB Function1/1(match_point_index_set) -> Cartesian2Frenet2/9(proj_match_point_index_set)
  [index2s] -> Cartesian2Frenet2/14(index2s)
  MATLAB Function1/3(proj_y_set) -> Cartesian2Frenet2/11(proj_y_set)
  Cartesian2Frenet2/1(Cartesian2FrenetOut) -> Bus Selector1/1
  [referenceline_kappa] -> MATLAB Function1/6(frenet_path_kappa)
  Bus Selector1/4 -> [dynamic_obs_l_dot_set_init]  "<l_dot_set>"
  [dynamic_obs_y_set_init] -> MATLAB Function1/2(y_set)
  [dynamic_obs_vx_set_init] -> Cartesian2Frenet2/3(vx_set)
  Bus Selector1/2 -> [dynamic_obs_l_set_init]  "<l_set>"
  MATLAB Function1/2(proj_x_set) -> Cartesian2Frenet2/10(proj_x_set)
  Ground4/1 -> Cartesian2Frenet2/5(ax_set)
  Bus Selector1/1 -> [dynamic_obs_s_set_init]  "<s_set>"
  [referenceline_x] -> Cartesian2Frenet2/7(frenet_path_x)
  [obs_heading_set_final] -> MATLAB Function/3(obs_heading_set_gcs)
  [obs_velocity_set_final] -> MATLAB Function/4(obs_velocity_set_gcs)
  [dynamic_obs_x_set] -> dynamic_obs_x_set/1
  [dynamic_obs_y_set] -> dynamic_obs_y_set/1
  [dynamic_obs_vx_set] -> dynamic_obs_vx_set/1
  [dynamic_obs_vy_set] -> dynamic_obs_vy_set/1
  [static_obs_l_set] -> static_obs_l_set/1
  [static_obs_s_set] -> static_obs_s_set/1
  index2s/1 -> [index2s]
  referenceline_kappa/1 -> [referenceline_kappa]
  referenceline_heading/1 -> [referenceline_heading]
  referenceline_y/1 -> [referenceline_y]
  referenceline_x/1 -> [referenceline_x]
  obs_heading_set_gcs/1 -> [obs_heading_set_gcs]
  obs_velocity_set_gcs/1 -> [obs_velocity_set_gcs]
  obs_y_set_gcs/1 -> [obs_y_set_gcs]
  obs_x_set_gcs/1 -> [obs_x_set_gcs]
  host_heading_xy/1 -> [host_heading_xy]
  host_y/1 -> [host_y]
  host_x/1 -> [host_x]
  [static_obs_y_set] -> Cartesian2Frenet1/2(y_set)
  MATLAB Function/2(static_obs_y_set) -> [static_obs_y_set]
  [static_obs_x_set] -> MATLAB Function2/1(x_set)
  Cartesian2Frenet1/1(Cartesian2FrenetOut) -> Bus Selector5/1
  [obs_y_set_gcs] -> obs filter/5(obs_y_set_gcs)
  [host_x] -> obs filter/1(host_x)
  MATLAB Function2/1(match_point_index_set) -> Cartesian2Frenet1/9(proj_match_point_index_set)
  MATLAB Function/4(dynamic_obs_y_set) -> [dynamic_obs_y_set_init]
  MATLAB Function2/3(proj_y_set) -> Cartesian2Frenet1/11(proj_y_set)
  Ground/1 -> Cartesian2Frenet1/3(vx_set)
  MATLAB Function2/2(proj_x_set) -> Cartesian2Frenet1/10(proj_x_set)
  MATLAB Function/3(dynamic_obs_x_set) -> [dynamic_obs_x_set_init]
  Bus Selector5/1 -> [static_obs_s_set_init]  "<s_set>"
  obs filter/2(obs_y_set_final) -> [obs_y_set_final]
  [referenceline_heading] -> MATLAB Function2/5(frenet_path_heading)
  Bus Selector5/2 -> [static_obs_l_set_init]  "<l_set>"
  [host_y] -> obs filter/2(host_y)
  [obs_velocity_set_gcs] -> obs filter/6(obs_velocity_set_gcs)
  [obs_x_set_final] -> MATLAB Function/1(obs_x_set_gcs)
  Ground1/1 -> Cartesian2Frenet1/4(vy_set)
  [referenceline_x] -> Cartesian2Frenet1/7(frenet_path_x)
  [static_obs_y_set] -> MATLAB Function2/2(y_set)
  [static_obs_x_set] -> Cartesian2Frenet1/1(x_set)
  [referenceline_kappa] -> MATLAB Function2/6(frenet_path_kappa)
  [obs_heading_set_gcs] -> obs filter/7(obs_heading_set_gcs)
  MATLAB Function/1(static_obs_x_set) -> [static_obs_x_set]
  obs filter/3(obs_velocity_set_final) -> [obs_velocity_set_final]
  [referenceline_y] -> MATLAB Function2/4(frenet_path_y)
  MATLAB Function/6(dynamic_obs_vy_set) -> [dynamic_obs_vy_set_init]
  [obs_y_set_final] -> MATLAB Function/2(obs_y_set_gcs)
  MATLAB Function/5(dynamic_obs_vx_set) -> [dynamic_obs_vx_set_init]
  [host_heading_xy] -> obs filter/3(host_heading_xy)
  obs filter/4(obs_heading_set_final) -> [obs_heading_set_final]
  obs filter/1(obs_x_set_final) -> [obs_x_set_final]
  Ground2/1 -> Cartesian2Frenet1/5(ax_set)
  [referenceline_x] -> MATLAB Function2/3(frenet_path_x)
  MATLAB Function2/4(proj_heading_set) -> Cartesian2Frenet1/12(proj_heading_set)
  MATLAB Function2/5(proj_kappa_set) -> Cartesian2Frenet1/13(proj_kappa_set)
  [referenceline_y] -> Cartesian2Frenet1/8(frenet_path_y)
  [index2s] -> Cartesian2Frenet1/14(index2s)
  [obs_x_set_gcs] -> obs filter/4(obs_x_set_gcs)
  Ground3/1 -> Cartesian2Frenet1/6(ay_set)

== system formation_planner_exp_cs/Global_Planner/Path planning/Planner Car1/path decision task ==
  static_obs_s_set : Inport
  static_obs_l_set : Inport  Port=2
  plan_start_s : Inport  Port=3
  plan_start_l : Inport  Port=4
  plan_start_dl : Inport  Port=5
  plan_start_ddl : Inport  Port=6
  dp_cost_collision : Inport  Port=7
  dp_cost_dl : Inport  Port=8
  dp_cost_ddl : Inport  Port=9
  dp_cost_dddl : Inport  Port=10
  dp_cost_ref : Inport  Port=11
  dp_row : Inport  Port=12
  dp_col : Inport  Port=13
  dp_sample_s : Inport  Port=14
  dp_sample_l : Inport  Port=15
  increase DP path nodes : MATLAB Function  TreatAsAtomicUnit=on
  path decision with dynamic planning(dp) : MATLAB Function  TreatAsAtomicUnit=on
  dp_path_s_final : Outport
  dp_path_l_final : Outport  Port=2
  dp_path_dl_final : Outport  Port=3
  dp_path_ddl_final : Outport  Port=4
  wires:
  dp_cost_collision/1 -> [dp_cost_collision]
  dp_sample_s/1 -> [dp_sample_s]
  dp_sample_l/1 -> [dp_sample_l]
  dp_col/1 -> [dp_col]
  dp_row/1 -> [dp_row]
  dp_cost_ref/1 -> [dp_cost_ref]
  dp_cost_dddl/1 -> [dp_cost_dddl]
  dp_cost_ddl/1 -> [dp_cost_ddl]
  dp_cost_dl/1 -> [dp_cost_dl]
  [dp_sample_l] -> path decision with dynamic planning(dp)/15(sample_l)
  [dp_sample_s] -> path decision with dynamic planning(dp)/14(sample_s)
  [dp_col] -> path decision with dynamic planning(dp)/13(col)
  [dp_row] -> path decision with dynamic planning(dp)/12(row)
  [dp_cost_ref] -> path decision with dynamic planning(dp)/11(w_cost_ref)
  [dp_cost_dddl] -> path decision with dynamic planning(dp)/10(w_cost_smooth_dddl)
  [dp_cost_ddl] -> path decision with dynamic planning(dp)/9(w_cost_smooth_ddl)
  [dp_cost_dl] -> path decision with dynamic planning(dp)/8(w_cost_smooth_dl)
  [dp_cost_collision] -> path decision with dynamic planning(dp)/7(w_cost_collision)
  [dp_path_ddl_final] -> dp_path_ddl_final/1
  [dp_path_dl_final] -> dp_path_dl_final/1
  [dp_path_l_final] -> dp_path_l_final/1
  [dp_path_s_final] -> dp_path_s_final/1
  plan_start_ddl/1 -> [plan_start_ddl]
  plan_start_dl/1 -> [plan_start_dl]
  plan_start_l/1 -> [plan_start_l]
  plan_start_s/1 -> [plan_start_s]
  static_obs_l_set/1 -> [static_obs_l_set]
  static_obs_s_set/1 -> [static_obs_s_set]
  [dp_path_s_init] -> increase DP path nodes/1(dp_path_s_init)
  [dp_path_l_init] -> increase DP path nodes/2(dp_path_l_init)
  [plan_start_s] -> increase DP path nodes/3(plan_start_s)
  [plan_start_dl] -> path decision with dynamic planning(dp)/5(plan_start_dl)
  [plan_start_ddl] -> increase DP path nodes/6(plan_start_ddl)
  [plan_start_l] -> increase DP path nodes/4(plan_start_l)
  path decision with dynamic planning(dp)/2(dp_path_l) -> [dp_path_l_init]
  increase DP path nodes/3(dp_path_dl_final) -> [dp_path_dl_final]
  increase DP path nodes/1(dp_path_s_final) -> [dp_path_s_final]
  increase DP path nodes/4(dp_path_ddl_final) -> [dp_path_ddl_final]
  [plan_start_dl] -> increase DP path nodes/5(plan_start_dl)
  [static_obs_s_set] -> path decision with dynamic planning(dp)/1(obs_s_set)
  [plan_start_l] -> path decision with dynamic planning(dp)/4(plan_start_l)
  [plan_start_ddl] -> path decision with dynamic planning(dp)/6(plan_start_dll)
  [static_obs_l_set] -> path decision with dynamic planning(dp)/2(obs_l_set)
  increase DP path nodes/2(dp_path_l_final) -> [dp_path_l_final]
  path decision with dynamic planning(dp)/1(dp_path_s) -> [dp_path_s_init]
  [plan_start_s] -> path decision with dynamic planning(dp)/3(plan_start_s)

== system formation_planner_exp_cs/Global_Planner/Path planning/Planner Car1/path planning task ==
  dp_path_s_final : Inport
  dp_path_l_final : Inport  Port=2
  static_obs_s_set : Inport  Port=3
  static_obs_l_set : Inport  Port=4
  plan_start_s : Inport  Port=5
  plan_start_l : Inport  Port=6
  plan_start_dl : Inport  Port=7
  plan_start_ddl : Inport  Port=8
  qp_cost_l : Inport  Port=9
  qp_cost_dl : Inport  Port=10
  qp_cost_ddl : Inport  Port=11
  qp_cost_dddl : Inport  Port=12
  qp_cost_centre : Inport  Port=13
  qp_cost_endl : Inport  Port=14
  qp_cost_end_dl : Inport  Port=15
  qp_cost_end_ddl : Inport  Port=16
  host_d1 : Inport  Port=17
  host_d2 : Inport  Port=18
  host_w : Inport  Port=19
  delta_dl_max : Inport  Port=20
  delta_ddl_max : Inport  Port=21
  Constant10 : Constant  Value=5
  Constant11 : Constant  Value=3
  MATLAB Function : MATLAB Function  TreatAsAtomicUnit=on
  generate convex space : MATLAB Function  TreatAsAtomicUnit=on
  path planning with quadratic programming (qp) : MATLAB Function  TreatAsAtomicUnit=on
  qp_path_s_final : Outport
  qp_path_l_final : Outport  Port=2
  qp_path_dl_final : Outport  Port=3
  qp_path_ddl_final : Outport  Port=4
  wires:
  path planning with quadratic programming (qp)/4(qp_path_ddl) -> [qp_path_ddl]
  path planning with quadratic programming (qp)/3(qp_path_dl) -> [qp_path_dl]
  path planning with quadratic programming (qp)/2(qp_path_l) -> [qp_path_l]
  path planning with quadratic programming (qp)/1(qp_path_s) -> [qp_path_s]
  [qp_path_ddl_final] -> qp_path_ddl_final/1
  [qp_path_dl_final] -> qp_path_dl_final/1
  [qp_path_l_final] -> qp_path_l_final/1
  [qp_path_s_final] -> qp_path_s_final/1
  [qp_path_l] -> MATLAB Function/2(qp_path_l)
  MATLAB Function/4(qp_path_ddl_final) -> [qp_path_ddl_final]
  [qp_path_dl] -> MATLAB Function/3(qp_path_dl)
  MATLAB Function/2(qp_path_l_final) -> [qp_path_l_final]
  [qp_path_ddl] -> MATLAB Function/4(qp_path_ddl)
  [qp_path_s] -> MATLAB Function/1(qp_path_s)
  MATLAB Function/3(qp_path_dl_final) -> [qp_path_dl_final]
  MATLAB Function/1(qp_path_s_final) -> [qp_path_s_final]
  [plan_start_s] -> path planning with quadratic programming (qp)/14(plan_start_s)
  plan_start_s/1 -> [plan_start_s]
  delta_ddl_max/1 -> [delta_ddl_max]
  delta_dl_max/1 -> [delta_dl_max]
  [delta_ddl_max] -> path planning with quadratic programming (qp)/19(delta_ddl_max)
  [delta_dl_max] -> path planning with quadratic programming (qp)/18(delta_dl_max)
  host_w/1 -> [host_w]
  host_d2/1 -> [host_d2]
  host_d1/1 -> [host_d1]
  qp_cost_end_ddl/1 -> [qp_cost_end_ddl]
  qp_cost_end_dl/1 -> [qp_cost_end_dl]
  qp_cost_endl/1 -> [qp_cost_endl]
  qp_cost_centre/1 -> [qp_cost_centre]
  qp_cost_dddl/1 -> [qp_cost_dddl]
  qp_cost_ddl/1 -> [qp_cost_ddl]
  qp_cost_dl/1 -> [qp_cost_dl]
  qp_cost_l/1 -> [qp_cost_l]
  [host_w] -> path planning with quadratic programming (qp)/13(host_w)
  [host_d2] -> path planning with quadratic programming (qp)/12(host_d2)
  [host_d1] -> path planning with quadratic programming (qp)/11(host_d1)
  [qp_cost_end_ddl] -> path planning with quadratic programming (qp)/10(w_cost_end_ddl)
  [qp_cost_end_dl] -> path planning with quadratic programming (qp)/9(w_cost_end_dl)
  [qp_cost_endl] -> path planning with quadratic programming (qp)/8(w_cost_end_l)
  [qp_cost_centre] -> path planning with quadratic programming (qp)/7(w_cost_centre)
  [qp_cost_dddl] -> path planning with quadratic programming (qp)/6(w_cost_dddl)
  [qp_cost_ddl] -> path planning with quadratic programming (qp)/5(w_cost_ddl)
  [qp_cost_dl] -> path planning with quadratic programming (qp)/4(w_cost_dl)
  [qp_cost_l] -> path planning with quadratic programming (qp)/3(w_cost_l)
  plan_start_ddl/1 -> [plan_start_ddl]
  plan_start_dl/1 -> [plan_start_dl]
  plan_start_l/1 -> [plan_start_l]
  static_obs_l_set/1 -> [static_obs_l_set]
  static_obs_s_set/1 -> [static_obs_s_set]
  dp_path_l_final/1 -> [dp_path_l_final]
  dp_path_s_final/1 -> [dp_path_s_final]
  [plan_start_ddl] -> path planning with quadratic programming (qp)/17(plan_start_ddl)
  [l_min] -> path planning with quadratic programming (qp)/1(l_min)
  [l_max] -> path planning with quadratic programming (qp)/2(l_max)
  [plan_start_dl] -> path planning with quadratic programming (qp)/16(plan_start_dl)
  [dp_path_l_final] -> generate convex space/2(dp_path_l)
  [static_obs_s_set] -> generate convex space/3(static_obs_s_set)
  generate convex space/1(l_min) -> [l_min]
  [plan_start_l] -> path planning with quadratic programming (qp)/15(plan_start_l)
  [dp_path_s_final] -> generate convex space/1(dp_path_s)
  [static_obs_l_set] -> generate convex space/4(static_obs_l_set)
  Constant10/1 -> generate convex space/5(static_obs_length)
  Constant11/1 -> generate convex space/6(static_obs_width)
  generate convex space/2(l_max) -> [l_max]

== system formation_planner_exp_cs/Global_Planner/Path planning/Planner Car2/Cartesian2Frenet ==
  x_set : Inport
  y_set : Inport  Port=2
  vx_set : Inport  Port=3
  vy_set : Inport  Port=4
  ax_set : Inport  Port=5
  ay_set : Inport  Port=6
  frenet_path_x : Inport  Port=7
  frenet_path_y : Inport  Port=8
  proj_match_point_index_set : Inport  Port=9
  proj_x_set : Inport  Port=10
  proj_y_set : Inport  Port=11
  proj_heading_set : Inport  Port=12
  proj_kappa_set : Inport  Port=13
  index2s : Inport  Port=14
  Bus Creator : BusCreator  Inputs=8
  MATLAB Function : MATLAB Function  TreatAsAtomicUnit=on
  MATLAB Function1 : MATLAB Function  TreatAsAtomicUnit=on
  MATLAB Function2 : MATLAB Function  TreatAsAtomicUnit=on
  Cartesian2FrenetOut : Outport
  wires:
  Bus Creator/1 -> Cartesian2FrenetOut/1
  [ddl_set] -> Bus Creator/8  "ddl_set"
  [l_dot2_set] -> Bus Creator/7  "l_dot2_set"
  [s_dot2_set] -> Bus Creator/6  "s_dot2_set"
  [dl_set] -> Bus Creator/5  "dl_set"
  [l_dot_set] -> Bus Creator/4  "l_dot_set"
  [s_dot_set] -> Bus Creator/3  "s_dot_set"
  [l_set] -> Bus Creator/2  "l_set"
  [s_set] -> Bus Creator/1  "s_set"
  MATLAB Function2/3(ddl_set) -> [ddl_set]
  MATLAB Function2/2(l_dot2_set) -> [l_dot2_set]
  MATLAB Function2/1(s_dot2_set) -> [s_dot2_set]
  [dl_set] -> MATLAB Function2/7(dl_set)
  [s_dot_set] -> MATLAB Function2/6(s_dot_set)
  MATLAB Function1/3(dl_set) -> [dl_set]
  MATLAB Function1/2(l_dot_set) -> [l_dot_set]
  MATLAB Function1/1(s_dot_set) -> [s_dot_set]
  [l_set] -> MATLAB Function2/5(l_set)
  [proj_kappa_set] -> MATLAB Function2/4(proj_kappa_set)
  [proj_heading_set] -> MATLAB Function2/3(proj_heading_set)
  [ay_set] -> MATLAB Function2/2(ay_set)
  [ax_set] -> MATLAB Function2/1(ax_set)
  [proj_kappa_set] -> MATLAB Function1/5(proj_kappa_set)
  [proj_heading_set] -> MATLAB Function1/4(proj_heading_set)
  [vy_set] -> MATLAB Function1/3(vy_set)
  [vx_set] -> MATLAB Function1/2(vx_set)
  [l_set] -> MATLAB Function1/1(l_set)
  MATLAB Function/2(l_set) -> [l_set]
  MATLAB Function/1(s_set) -> [s_set]
  [index2s] -> MATLAB Function/9(index2s)
  [proj_heading_set] -> MATLAB Function/7(proj_heading_set)
  [proj_y_set] -> MATLAB Function/6(proj_y_set)
  [proj_match_point_index_set] -> MATLAB Function/8(proj_match_point_index_set)
  [proj_x_set] -> MATLAB Function/5(proj_x_set)
  [frenet_path_y] -> MATLAB Function/4(frenet_path_y)
  [frenet_path_x] -> MATLAB Function/3(frenet_path_x)
  [y_set] -> MATLAB Function/2(y_set)
  [x_set] -> MATLAB Function/1(x_set)
  index2s/1 -> [index2s]
  proj_kappa_set/1 -> [proj_kappa_set]
  proj_heading_set/1 -> [proj_heading_set]
  proj_y_set/1 -> [proj_y_set]
  proj_x_set/1 -> [proj_x_set]
  proj_match_point_index_set/1 -> [proj_match_point_index_set]
  frenet_path_y/1 -> [frenet_path_y]
  frenet_path_x/1 -> [frenet_path_x]
  ay_set/1 -> [ay_set]
  ax_set/1 -> [ax_set]
  vy_set/1 -> [vy_set]
  vx_set/1 -> [vx_set]
  y_set/1 -> [y_set]
  x_set/1 -> [x_set]
